simulink model "restapi_slave_task"  (Simulink 3.00)
libraries: mathlib x1, analoglib x1

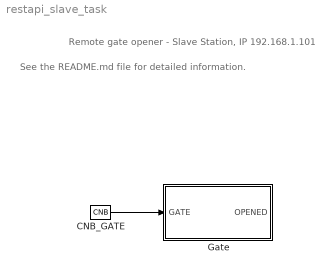
== system restapi_slave_task ==
  note: See the README.md file for detailed information.
  note: Remote gate opener - Slave Station, IP 192.168.1.101
  CNB_GATE : mathlib/CNB  YCN=off
  Gate : Subsystem
      mask Type: REX sequence
  wires:
  CNB_GATE/1 -> Gate/1(GATE)

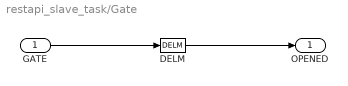
== system restapi_slave_task/Gate ==
  GATE : Inport  Port=1
  DELM : analoglib/DELM  del=5  nmax=100
  OPENED : Outport  Port=1
  wires:
  DELM/1 -> OPENED/1
  GATE/1 -> DELM/1
